simulink library "untitled"  (R2023b)
settings: Solver=VariableStepAuto  StartTime=0.0  StopTime=10.0  RelTol=1e-3
undefined symbols (not defined in the file): LowerUserTemp
settings Model: Creator=mueller.chris-it22  LastModifiedBy=mueller.chris-it22

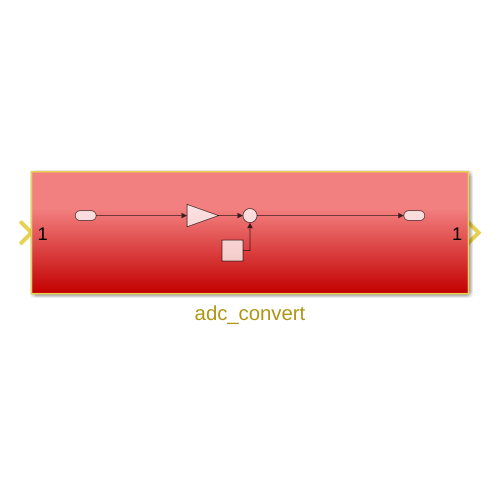
[thumbnail: Simulink's stored preview of the top-level diagram]
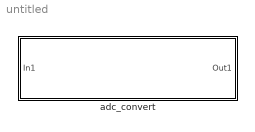
== system untitled ==
  adc_convert : Subsystem

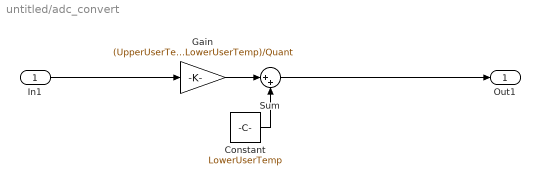
== system untitled/adc_convert ==
  In1 : Inport
  Constant : Constant  Value=LowerUserTemp  OutDataTypeStr=uint16
  Gain : Gain  Gain=(UpperUserTemp - LowerUserTemp)/Quant  OutDataTypeStr=uint16
  Sum : Sum  Inputs=|++
  Out1 : Outport
  wires:
  Gain/1 -> Sum/1
  In1/1 -> Gain/1
  Constant/1 -> Sum/2
  Sum/1 -> Out1/1
